simulink model "MCU_vectorControl_dsPIC33AK128MC106_MCLV_48V_300W_Float"  (R2024b)
settings: Solver=FixedStepDiscrete  StartTime=0.0  StopTime=10.0  FixedStep=50e-6  RelTol=1e-3  EnableMultiTasking=on
undefined symbols (not defined in the file or in its folder): A0, A4, ADC, B0, C10, C11, C6, C7, C8, control, D11, D12, DiscIntNeverNeededParam, inverter, Max, MaxPer, model, ms, NumBits1, NumBits2, P1, P17, P20, P39, P40, P41, P43, P44, P60, P61, Pin, PosRange1, PosRange2, PWM1_Trg1, Resol, s, Slope1, Slope2, us
libraries: simulink x35, MCHP_Blockset x22
(part 4 of 5)

== system MCU_vectorControl_dsPIC33AK128MC106_MCLV_48V_300W_Float/BOARD MCLV-48V-300W dsPIC33AK128MC106 MC DIM/ADC ==
  note: A5: IBUS
      | A7: VBUS
      | A11: Pot
  ADC HS 12b dsPICA1 : MCHP_Blockset/Analog IO/ADC HS 12b dsPICA  ADCREF=ADC 1 and ADC 2  ADC1_refChannel=0 (highest priority)  ADC2_refChannel=0 (highest priority)  ADC3_refChannel=Not used  ADC4_refChannel=Not used  ADC5_refChannel=Not used  CALRATE=once at startup  VREF_RNG=3.0V to 3.6V  BUFEN=off  info=0  SampleTime=1/Switching_Frequency  MCHP_PORT={ADC1_seq0.0}{ADC1A2}15:2:A2;{ADC2_seq0.0}{ADC2B0}15:2:B0;{ADC1_seq0.1}{ADC1B8}15:2:B8;{ADC2_seq0.1}{ADC2B9}15:2:B9;{ADC2_seq0.2}{ADC2A10}15:2:A10;{ADC1_seq0.0}{ADC1A2}15:2:A2;{ADC2_seq0.0}{ADC2B0}15:2:B0;{ADC1_seq0.1}{ADC1B8}15:2:B8;{ADC2_seq0.1}{ADC2B9}15:2:B9;{ADC2_seq0.2}{ADC2A10}15:2:A10;  MCHP_MASTERLINK=MCU_vectorControl_dsPIC33AK128MC106_MCLV_48V_300W_Flt/BOARD MCLV-48V-300W dsPIC33AK128MC106 MC DIM/Microchip Master  MCHP_CRC=34075787  ADC_Synchronisation=Triggered by custom source  ADC_Trig_TXT=PWM1_Trg1  ADC_TrigTimeStep=on  TrigSource_seq0_TXT=PWM1 adc trig 1  SampleTime_seq0_Tad_TXT="4.5 Tad  = 56.2ns  -  Rin < 5.2 kOhm"  ADC1_seq0_TXT=AD1 AN0 / A2 / Pin[12]  ADC1_seq0_align=Left aligned  ADC1_seq0_overSampling=x1 (12 bits)  ADC2_seq0_TXT=AD2 AN1 / B0 / Pin[20]  ADC2_seq0_align=Left aligned  ADC2_seq0_overSampling=x1 (12 bits)  ADC3_seq0_TXT="AD2 AN1 / B0 / Pin[20]  (L)"  ADC3_seq0_align=Right aligned  ADC3_seq0_overSampling=x1 (12 bits)  ADC4_seq0_TXT="AD2 AN1 / B0 / Pin[20]  (L)"  ADC4_seq0_align=Right aligned  ADC4_seq0_overSampling=x1 (12 bits)  ADC5_seq0_TXT="AD2 AN1 / B0 / Pin[20]  (L)"  ADC5_seq0_align=Right aligned  ADC5_seq0_overSampling=x1 (12 bits)  ADC1_seq0_1_TXT=AD1 AN11 / B8 / Pin[23]  ADC1_seq0_1_align=Left aligned  ADC1_seq0_1_overSampling=x1 (12 bits)  ADC2_seq0_1_TXT=AD2 AN10 / B9 / Pin[24]  ADC2_seq0_1_align=Left aligned  ADC2_seq0_1_overSampling=x1 (12 bits)  ADC3_seq0_1_TXT=Not Used  ADC3_seq0_1_align=Right aligned  ADC3_seq0_1_overSampling=x1 (12 bits)  ADC4_seq0_1_TXT=Not Used  ADC4_seq0_1_align=Right aligned  ADC4_seq0_1_overSampling=x1 (12 bits)  ADC5_seq0_1_TXT=Not Used  ADC5_seq0_1_align=Right aligned  ADC5_seq0_1_overSampling=x1 (12 bits)  ADC1_seq0_2_TXT=Not Used  ADC1_seq0_2_align=Right aligned  ADC1_seq0_2_overSampling=x1 (12 bits)  ADC2_seq0_2_TXT=AD2 AN7 / A10 / Pin[9]  ADC2_seq0_2_align=Left aligned  ADC2_seq0_2_overSampling=x1 (12 bits)  ADC3_seq0_2_TXT=Not Used  ADC3_seq0_2_align=Right aligned  ADC3_seq0_2_overSampling=x1 (12 bits)  ADC4_seq0_2_TXT=Not Used  ADC4_seq0_2_align=Right aligned  ADC4_seq0_2_overSampling=x1 (12 bits)  ADC5_seq0_2_TXT=Not Used  ADC5_seq0_2_align=Right aligned  ADC5_seq0_2_overSampling=x1 (12 bits)  ADC1_seq0_3_TXT=Not Used  ADC1_seq0_3_align=Right aligned  ADC1_seq0_3_overSampling=x1 (12 bits)  ADC2_seq0_3_TXT=Not Used  ADC2_seq0_3_align=Right aligned  ADC2_seq0_3_overSampling=x1 (12 bits)  ADC3_seq0_3_TXT=Not Used  ADC3_seq0_3_align=Right aligned  ADC3_seq0_3_overSampling=x1 (12 bits)  ADC4_seq0_3_TXT=Not Used  ADC4_seq0_3_align=Right aligned  ADC4_seq0_3_overSampling=x1 (12 bits)  ADC5_seq0_3_TXT=Not Used  ADC5_seq0_3_align=Right aligned  ADC5_seq0_3_overSampling=x1 (12 bits)  ADC1_seq0_4_TXT=Not Used  ADC1_seq0_4_align=Right aligned  ADC1_seq0_4_overSampling=x1 (12 bits)  ADC2_seq0_4_TXT=Not Used  ADC2_seq0_4_align=Right aligned  ADC2_seq0_4_overSampling=x1 (12 bits)  ADC3_seq0_4_TXT=Not Used  ADC3_seq0_4_align=Right aligned  ADC3_seq0_4_overSampling=x1 (12 bits)  ADC4_seq0_4_TXT=Not Used  ADC4_seq0_4_align=Right aligned  ADC4_seq0_4_overSampling=x1 (12 bits)  ADC5_seq0_4_TXT=Not Used  ADC5_seq0_4_align=Right aligned  ADC5_seq0_4_overSampling=x1 (12 bits)  ADC1_seq0_5_TXT=Not Used  ADC1_seq0_5_align=Right aligned  ADC1_seq0_5_overSampling=x1 (12 bits)  ADC2_seq0_5_TXT=Not Used  ADC2_seq0_5_align=Right aligned  ADC2_seq0_5_overSampling=x1 (12 bits)  ADC3_seq0_5_TXT=Not Used  ADC3_seq0_5_align=Right aligned  ADC3_seq0_5_overSampling=x1 (12 bits)  ADC4_seq0_5_TXT=Not Used  ADC4_seq0_5_align=Right aligned  ADC4_seq0_5_overSampling=x1 (12 bits)  ADC5_seq0_5_TXT=Not Used  ADC5_seq0_5_align=Right aligned  ADC5_seq0_5_overSampling=x1 (12 bits)  ADC_TRG2_ACCBRST_seq0=Burst - not interruptible  ADC1_NINSEL_seq0_TXT=Vss - single ended (unsigned)  ADC2_NINSEL_seq0_TXT=Vss - single ended (unsigned)  ADC3_NINSEL_seq0_TXT=Vss - single ended (unsigned)  ADC4_NINSEL_seq0_TXT=Vss - single ended (unsigned)  ADC5_NINSEL_seq0_TXT=Vss - single ended (unsigned)  TrigTimeStep_seq0=on  info_seq0=0  TrigSource_seq1_TXT=after previous sequence  SampleTime_seq1_Tad_TXT="0.5 Tad  = 6.25ns  -  Rin < 0 kOhm"  ADC1_seq1_TXT=Not Used  ADC1_seq1_align=Right aligned  ADC1_seq1_overSampling=x1 (12 bits)  ADC2_seq1_TXT=Not Used  ADC2_seq1_align=Right aligned  ADC2_seq1_overSampling=x1 (12 bits)  ADC3_seq1_TXT=Not Used  ADC3_seq1_align=Right aligned  ADC3_seq1_overSampling=x1 (12 bits)  ADC4_seq1_TXT=Not Used  ADC4_seq1_align=Right aligned  ADC4_seq1_overSampling=x1 (12 bits)  ADC5_seq1_TXT=Not Used  ADC5_seq1_align=Right aligned  ADC5_seq1_overSampling=x1 (12 bits)  ADC1_seq1_1_TXT=Not Used  ADC1_seq1_1_align=Right aligned  ADC1_seq1_1_overSampling=x1 (12 bits)  ADC2_seq1_1_TXT=Not Used  ADC2_seq1_1_align=Right aligned  ADC2_seq1_1_overSampling=x1 (12 bits)  ADC3_seq1_1_TXT=Not Used  ADC3_seq1_1_align=Right aligned  ADC3_seq1_1_overSampling=x1 (12 bits)  ADC4_seq1_1_TXT=Not Used  ADC4_seq1_1_align=Right aligned  ADC4_seq1_1_overSampling=x1 (12 bits)  ADC5_seq1_1_TXT=Not Used  ADC5_seq1_1_align=Right aligned  ADC5_seq1_1_overSampling=x1 (12 bits)  ADC1_seq1_2_TXT=Not Used  ADC1_seq1_2_align=Right aligned  ADC1_seq1_2_overSampling=x1 (12 bits)  ADC2_seq1_2_TXT=Not Used  ADC2_seq1_2_align=Right aligned  ADC2_seq1_2_overSampling=x1 (12 bits)  ADC3_seq1_2_TXT=Not Used  ADC3_seq1_2_align=Right aligned  ADC3_seq1_2_overSampling=x1 (12 bits)  ADC4_seq1_2_TXT=Not Used  ADC4_seq1_2_align=Right aligned  ADC4_seq1_2_overSampling=x1 (12 bits)  ADC5_seq1_2_TXT=Not Used  ADC5_seq1_2_align=Right aligned  ADC5_seq1_2_overSampling=x1 (12 bits)  ADC1_seq1_3_TXT=Not Used  ADC1_seq1_3_align=Right aligned  ADC1_seq1_3_overSampling=x1 (12 bits)  ADC2_seq1_3_TXT=Not Used  ADC2_seq1_3_align=Right aligned  ADC2_seq1_3_overSampling=x1 (12 bits)  ADC3_seq1_3_TXT=Not Used  ADC3_seq1_3_align=Right aligned  ADC3_seq1_3_overSampling=x1 (12 bits)  ADC4_seq1_3_TXT=Not Used  ADC4_seq1_3_align=Right aligned  ADC4_seq1_3_overSampling=x1 (12 bits)  ADC5_seq1_3_TXT=Not Used  ADC5_seq1_3_align=Right aligned  ADC5_seq1_3_overSampling=x1 (12 bits)  ADC1_seq1_4_TXT=Not Used  ADC1_seq1_4_align=Right aligned  ADC1_seq1_4_overSampling=x1 (12 bits)  ADC2_seq1_4_TXT=Not Used  ADC2_seq1_4_align=Right aligned  ADC2_seq1_4_overSampling=x1 (12 bits)  ADC3_seq1_4_TXT=Not Used  ADC3_seq1_4_align=Right aligned  ADC3_seq1_4_overSampling=x1 (12 bits)  ADC4_seq1_4_TXT=Not Used  ADC4_seq1_4_align=Right aligned  ADC4_seq1_4_overSampling=x1 (12 bits)  ADC5_seq1_4_TXT=Not Used  ADC5_seq1_4_align=Right aligned  ADC5_seq1_4_overSampling=x1 (12 bits)  ADC1_seq1_5_TXT=Not Used  ADC1_seq1_5_align=Right aligned  ADC1_seq1_5_overSampling=x1 (12 bits)  ADC2_seq1_5_TXT=Not Used  ADC2_seq1_5_align=Right aligned  ADC2_seq1_5_overSampling=x1 (12 bits)  ADC3_seq1_5_TXT=Not Used  ADC3_seq1_5_align=Right aligned  ADC3_seq1_5_overSampling=x1 (12 bits)  ADC4_seq1_5_TXT=Not Used  ADC4_seq1_5_align=Right aligned  ADC4_seq1_5_overSampling=x1 (12 bits)  ADC5_seq1_5_TXT=Not Used  ADC5_seq1_5_align=Right aligned  ADC5_seq1_5_overSampling=x1 (12 bits)  ADC_TRG2_ACCBRST_seq1=Burst - not interruptible  ADC1_NINSEL_seq1_TXT=Vss - single ended (unsigned)  ADC2_NINSEL_seq1_TXT=Vss - single ended (unsigned)  ADC3_NINSEL_seq1_TXT=Vss - single ended (unsigned)  ADC4_NINSEL_seq1_TXT=Vss - single ended (unsigned)  ADC5_NINSEL_seq1_TXT=Vss - single ended (unsigned)  TrigTimeStep_seq1=off  info_seq1=0  TrigSource_seq2_TXT=after previous sequence  SampleTime_seq2_Tad_TXT="0.5 Tad  = 6.25ns  -  Rin < 0 kOhm"  ADC1_seq2_TXT=Not Used  ADC1_seq2_align=Right aligned  ADC1_seq2_overSampling=x1 (12 bits)  ADC2_seq2_TXT=Not Used  ADC2_seq2_align=Right aligned  ADC2_seq2_overSampling=x1 (12 bits)  ADC3_seq2_TXT=Not Used  ADC3_seq2_align=Right aligned  ADC3_seq2_overSampling=x1 (12 bits)  ADC4_seq2_TXT=Not Used  ADC4_seq2_align=Right aligned  ADC4_seq2_overSampling=x1 (12 bits)  ADC5_seq2_TXT=Not Used  ADC5_seq2_align=Right aligned  ADC5_seq2_overSampling=x1 (12 bits)  ADC1_seq2_1_TXT=Not Used  ADC1_seq2_1_align=Right aligned  ADC1_seq2_1_overSampling=x1 (12 bits)  ADC2_seq2_1_TXT=Not Used  ADC2_seq2_1_align=Right aligned  ADC2_seq2_1_overSampling=x1 (12 bits)  ADC3_seq2_1_TXT=Not Used  ADC3_seq2_1_align=Right aligned  ADC3_seq2_1_overSampling=x1 (12 bits)  ADC4_seq2_1_TXT=Not Used  ADC4_seq2_1_align=Right aligned  ADC4_seq2_1_overSampling=x1 (12 bits)  ADC5_seq2_1_TXT=Not Used  ADC5_seq2_1_align=Right aligned  ADC5_seq2_1_overSampling=x1 (12 bits)  ADC1_seq2_2_TXT=Not Used  ADC1_seq2_2_align=Right aligned  ADC1_seq2_2_overSampling=x1 (12 bits)  ADC2_seq2_2_TXT=Not Used  ADC2_seq2_2_align=Right aligned  ADC2_seq2_2_overSampling=x1 (12 bits)  ADC3_seq2_2_TXT=Not Used  ADC3_seq2_2_align=Right aligned  ADC3_seq2_2_overSampling=x1 (12 bits)  ADC4_seq2_2_TXT=Not Used  ADC4_seq2_2_align=Right aligned  ADC4_seq2_2_overSampling=x1 (12 bits)  ADC5_seq2_2_TXT=Not Used  ADC5_seq2_2_align=Right aligned  ADC5_seq2_2_overSampling=x1 (12 bits)  ADC1_seq2_3_TXT=Not Used  ADC1_seq2_3_align=Right aligned  ADC1_seq2_3_overSampling=x1 (12 bits)  ADC2_seq2_3_TXT=Not Used  ADC2_seq2_3_align=Right aligned  ADC2_seq2_3_overSampling=x1 (12 bits)  ADC3_seq2_3_TXT=Not Used  ADC3_seq2_3_align=Right aligned  ADC3_seq2_3_overSampling=x1 (12 bits)  ADC4_seq2_3_TXT=Not Used  ADC4_seq2_3_align=Right aligned  ADC4_seq2_3_overSampling=x1 (12 bits)  ADC5_seq2_3_TXT=Not Used  ADC5_seq2_3_align=Right aligned  ADC5_seq2_3_overSampling=x1 (12 bits)  ADC1_seq2_4_TXT=Not Used  ADC1_seq2_4_align=Right aligned  ADC1_seq2_4_overSampling=x1 (12 bits)  ADC2_seq2_4_TXT=Not Used  ADC2_seq2_4_align=Right aligned  ADC2_seq2_4_overSampling=x1 (12 bits)  ADC3_seq2_4_TXT=Not Used  ADC3_seq2_4_align=Right aligned  ADC3_seq2_4_overSampling=x1 (12 bits)  ADC4_seq2_4_TXT=Not Used  ADC4_seq2_4_align=Right aligned  ADC4_seq2_4_overSampling=x1 (12 bits)  ADC5_seq2_4_TXT=Not Used  ADC5_seq2_4_align=Right aligned  ADC5_seq2_4_overSampling=x1 (12 bits)  ADC1_seq2_5_TXT=Not Used  ADC1_seq2_5_align=Right aligned  ADC1_seq2_5_overSampling=x1 (12 bits)  ADC2_seq2_5_TXT=Not Used  ADC2_seq2_5_align=Right aligned  ADC2_seq2_5_overSampling=x1 (12 bits)  ADC3_seq2_5_TXT=Not Used  ADC3_seq2_5_align=Right aligned  ADC3_seq2_5_overSampling=x1 (12 bits)  ADC4_seq2_5_TXT=Not Used  ADC4_seq2_5_align=Right aligned  ADC4_seq2_5_overSampling=x1 (12 bits)  ADC5_seq2_5_TXT=Not Used  ADC5_seq2_5_align=Right aligned  ADC5_seq2_5_overSampling=x1 (12 bits)  ADC_TRG2_ACCBRST_seq2=Burst - not interruptible  ADC1_NINSEL_seq2_TXT=Vss - single ended (unsigned)  ADC2_NINSEL_seq2_TXT=Vss - single ended (unsigned)  ADC3_NINSEL_seq2_TXT=Vss - single ended (unsigned)  ADC4_NINSEL_seq2_TXT=Vss - single ended (unsigned)  ADC5_NINSEL_seq2_TXT=Vss - single ended (unsigned)  TrigTimeStep_seq2=off  info_seq2=0  TrigSource_seq3_TXT=after previous sequence  SampleTime_seq3_Tad_TXT="0.5 Tad  = 6.25ns  -  Rin < 0 kOhm"  ADC1_seq3_TXT=Not Used  ADC1_seq3_align=Right aligned  ADC1_seq3_overSampling=x1 (12 bits)  ADC2_seq3_TXT=Not Used  ADC2_seq3_align=Right aligned  ADC2_seq3_overSampling=x1 (12 bits)  ADC3_seq3_TXT=Not Used  ADC3_seq3_align=Right aligned  ADC3_seq3_overSampling=x1 (12 bits)  ADC4_seq3_TXT=Not Used  ADC4_seq3_align=Right aligned  ADC4_seq3_overSampling=x1 (12 bits)  ADC5_seq3_TXT=Not Used  ADC5_seq3_align=Right aligned  ADC5_seq3_overSampling=x1 (12 bits)  ADC1_seq3_1_TXT=Not Used  ADC1_seq3_1_align=Right aligned  ADC1_seq3_1_overSampling=x1 (12 bits)  ADC2_seq3_1_TXT=Not Used  ADC2_seq3_1_align=Right aligned  ADC2_seq3_1_overSampling=x1 (12 bits)  ADC3_seq3_1_TXT=Not Used  ADC3_seq3_1_align=Right aligned  ADC3_seq3_1_overSampling=x1 (12 bits)  ADC4_seq3_1_TXT=Not Used  ADC4_seq3_1_align=Right aligned  ADC4_seq3_1_overSampling=x1 (12 bits)  ADC5_seq3_1_TXT=Not Used  ADC5_seq3_1_align=Right aligned  ADC5_seq3_1_overSampling=x1 (12 bits)  ADC1_seq3_2_TXT=Not Used  ADC1_seq3_2_align=Right aligned  ADC1_seq3_2_overSampling=x1 (12 bits)  ADC2_seq3_2_TXT=Not Used  ADC2_seq3_2_align=Right aligned  ADC2_seq3_2_overSampling=x1 (12 bits)  ADC3_seq3_2_TXT=Not Used  ADC3_seq3_2_align=Right aligned  ADC3_seq3_2_overSampling=x1 (12 bits)  ADC4_seq3_2_TXT=Not Used  ADC4_seq3_2_align=Right aligned  ADC4_seq3_2_overSampling=x1 (12 bits)  ADC5_seq3_2_TXT=Not Used  ADC5_seq3_2_align=Right aligned  ADC5_seq3_2_overSampling=x1 (12 bits)  ADC1_seq3_3_TXT=Not Used  ADC1_seq3_3_align=Right aligned  ADC1_seq3_3_overSampling=x1 (12 bits)  ADC2_seq3_3_TXT=Not Used  ADC2_seq3_3_align=Right aligned  ADC2_seq3_3_overSampling=x1 (12 bits)  ADC3_seq3_3_TXT=Not Used  ADC3_seq3_3_align=Right aligned  ADC3_seq3_3_overSampling=x1 (12 bits)  ADC4_seq3_3_TXT=Not Used  ADC4_seq3_3_align=Right aligned  ADC4_seq3_3_overSampling=x1 (12 bits)  ADC5_seq3_3_TXT=Not Used  ADC5_seq3_3_align=Right aligned  ADC5_seq3_3_overSampling=x1 (12 bits)  ADC1_seq3_4_TXT=Not Used  ADC1_seq3_4_align=Right aligned  ADC1_seq3_4_overSampling=x1 (12 bits)  ADC2_seq3_4_TXT=Not Used  ADC2_seq3_4_align=Right aligned  ADC2_seq3_4_overSampling=x1 (12 bits)  ADC3_seq3_4_TXT=Not Used  ADC3_seq3_4_align=Right aligned  ADC3_seq3_4_overSampling=x1 (12 bits)  ADC4_seq3_4_TXT=Not Used  ADC4_seq3_4_align=Right aligned  ADC4_seq3_4_overSampling=x1 (12 bits)  ADC5_seq3_4_TXT=Not Used  ADC5_seq3_4_align=Right aligned  ADC5_seq3_4_overSampling=x1 (12 bits)  ADC1_seq3_5_TXT=Not Used  ADC1_seq3_5_align=Right aligned  ADC1_seq3_5_overSampling=x1 (12 bits)  ADC2_seq3_5_TXT=Not Used  ADC2_seq3_5_align=Right aligned  ADC2_seq3_5_overSampling=x1 (12 bits)  ADC3_seq3_5_TXT=Not Used  ADC3_seq3_5_align=Right aligned  ADC3_seq3_5_overSampling=x1 (12 bits)  ADC4_seq3_5_TXT=Not Used  ADC4_seq3_5_align=Right aligned  ADC4_seq3_5_overSampling=x1 (12 bits)  ADC5_seq3_5_TXT=Not Used  ADC5_seq3_5_align=Right aligned  ADC5_seq3_5_overSampling=x1 (12 bits)  ADC_TRG2_ACCBRST_seq3=Burst - not interruptible  ADC1_NINSEL_seq3_TXT=Vss - single ended (unsigned)  ADC2_NINSEL_seq3_TXT=Vss - single ended (unsigned)  ADC3_NINSEL_seq3_TXT=Vss - single ended (unsigned)  ADC4_NINSEL_seq3_TXT=Vss - single ended (unsigned)  ADC5_NINSEL_seq3_TXT=Vss - single ended (unsigned)  TrigTimeStep_seq3=off  info_seq3=0  TrigSource_seq4_TXT=after previous sequence  SampleTime_seq4_Tad_TXT="0.5 Tad  = 6.25ns  -  Rin < 0 kOhm"  ADC1_seq4_TXT=Not Used  ADC1_seq4_align=Right aligned  ADC1_seq4_overSampling=x1 (12 bits)  ADC2_seq4_TXT=Not Used  ADC2_seq4_align=Right aligned  ADC2_seq4_overSampling=x1 (12 bits)  ADC3_seq4_TXT=Not Used  ADC3_seq4_align=Right aligned  ADC3_seq4_overSampling=x1 (12 bits)  ADC4_seq4_TXT=Not Used  ADC4_seq4_align=Right aligned  ADC4_seq4_overSampling=x1 (12 bits)  ADC5_seq4_TXT=Not Used  ADC5_seq4_align=Right aligned  ADC5_seq4_overSampling=x1 (12 bits)  ADC1_seq4_1_TXT=Not Used  ADC1_seq4_1_align=Right aligned  ADC1_seq4_1_overSampling=x1 (12 bits)  ADC2_seq4_1_TXT=Not Used  ADC2_seq4_1_align=Right aligned  ADC2_seq4_1_overSampling=x1 (12 bits)  ADC3_seq4_1_TXT=Not Used  ADC3_seq4_1_align=Right aligned  ADC3_seq4_1_overSampling=x1 (12 bits)  ADC4_seq4_1_TXT=Not Used  ADC4_seq4_1_align=Right aligned  ADC4_seq4_1_overSampling=x1 (12 bits)  ADC5_seq4_1_TXT=Not Used  ADC5_seq4_1_align=Right aligned  ADC5_seq4_1_overSampling=x1 (12 bits)  ADC1_seq4_2_TXT=Not Used  ADC1_seq4_2_align=Right aligned  ADC1_seq4_2_overSampling=x1 (12 bits)  ADC2_seq4_2_TXT=Not Used  ADC2_seq4_2_align=Right aligned  ADC2_seq4_2_overSampling=x1 (12 bits)  ADC3_seq4_2_TXT=Not Used  ADC3_seq4_2_align=Right aligned  ADC3_seq4_2_overSampling=x1 (12 bits)  ADC4_seq4_2_TXT=Not Used  ADC4_seq4_2_align=Right aligned  ADC4_seq4_2_overSampling=x1 (12 bits)  ADC5_seq4_2_TXT=Not Used  ADC5_seq4_2_align=Right aligned  ADC5_seq4_2_overSampling=x1 (12 bits)  ADC1_seq4_3_TXT=Not Used  ADC1_seq4_3_align=Right aligned  ADC1_seq4_3_overSampling=x1 (12 bits)  ADC2_seq4_3_TXT=Not Used  ADC2_seq4_3_align=Right aligned  ADC2_seq4_3_overSampling=x1 (12 bits)  ADC3_seq4_3_TXT=Not Used  ADC3_seq4_3_align=Right aligned  ADC3_seq4_3_overSampling=x1 (12 bits)  ADC4_seq4_3_TXT=Not Used  ADC4_seq4_3_align=Right aligned  ADC4_seq4_3_overSampling=x1 (12 bits)  ADC5_seq4_3_TXT=Not Used  ADC5_seq4_3_align=Right aligned  ADC5_seq4_3_overSampling=x1 (12 bits)  ADC1_seq4_4_TXT=Not Used  ADC1_seq4_4_align=Right aligned  ADC1_seq4_4_overSampling=x1 (12 bits)  ADC2_seq4_4_TXT=Not Used  ADC2_seq4_4_align=Right aligned  ADC2_seq4_4_overSampling=x1 (12 bits)  ADC3_seq4_4_TXT=Not Used  ADC3_seq4_4_align=Right aligned  ADC3_seq4_4_overSampling=x1 (12 bits)  ADC4_seq4_4_TXT=Not Used  ADC4_seq4_4_align=Right aligned  ADC4_seq4_4_overSampling=x1 (12 bits)  ADC5_seq4_4_TXT=Not Used  ADC5_seq4_4_align=Right aligned  ADC5_seq4_4_overSampling=x1 (12 bits)  ADC1_seq4_5_TXT=Not Used  ADC1_seq4_5_align=Right aligned  ADC1_seq4_5_overSampling=x1 (12 bits)  ADC2_seq4_5_TXT=Not Used  ADC2_seq4_5_align=Right aligned  ADC2_seq4_5_overSampling=x1 (12 bits)  ADC3_seq4_5_TXT=Not Used  ADC3_seq4_5_align=Right aligned  ADC3_seq4_5_overSampling=x1 (12 bits)  ADC4_seq4_5_TXT=Not Used  ADC4_seq4_5_align=Right aligned  ADC4_seq4_5_overSampling=x1 (12 bits)  ADC5_seq4_5_TXT=Not Used  ADC5_seq4_5_align=Right aligned  ADC5_seq4_5_overSampling=x1 (12 bits)  ADC_TRG2_ACCBRST_seq4=Burst - not interruptible  ADC1_NINSEL_seq4_TXT=Vss - single ended (unsigned)  ADC2_NINSEL_seq4_TXT=Vss - single ended (unsigned)  ADC3_NINSEL_seq4_TXT=Vss - single ended (unsigned)  ADC4_NINSEL_seq4_TXT=Vss - single ended (unsigned)  ADC5_NINSEL_seq4_TXT=Vss - single ended (unsigned)  TrigTimeStep_seq4=off  info_seq4=0  TrigSource_seq5_TXT=after previous sequence  SampleTime_seq5_Tad_TXT="0.5 Tad  = 6.25ns  -  Rin < 0 kOhm"  ADC1_seq5_TXT=Not Used  ADC1_seq5_align=Right aligned  ADC1_seq5_overSampling=x1 (12 bits)  ADC2_seq5_TXT=Not Used  ADC2_seq5_align=Right aligned  ADC2_seq5_overSampling=x1 (12 bits)  ADC3_seq5_TXT=Not Used  ADC3_seq5_align=Right aligned  ADC3_seq5_overSampling=x1 (12 bits)  ADC4_seq5_TXT=Not Used  ADC4_seq5_align=Right aligned  ADC4_seq5_overSampling=x1 (12 bits)  ADC5_seq5_TXT=Not Used  ADC5_seq5_align=Right aligned  ADC5_seq5_overSampling=x1 (12 bits)  ADC1_seq5_1_TXT=Not Used  ADC1_seq5_1_align=Right aligned  ADC1_seq5_1_overSampling=x1 (12 bits)  ADC2_seq5_1_TXT=Not Used  ADC2_seq5_1_align=Right aligned  ADC2_seq5_1_overSampling=x1 (12 bits)  ADC3_seq5_1_TXT=Not Used  ADC3_seq5_1_align=Right aligned  ADC3_seq5_1_overSampling=x1 (12 bits)  ADC4_seq5_1_TXT=Not Used  ADC4_seq5_1_align=Right aligned  ADC4_seq5_1_overSampling=x1 (12 bits)  ADC5_seq5_1_TXT=Not Used  ADC5_seq5_1_align=Right aligned  ADC5_seq5_1_overSampling=x1 (12 bits)  ADC1_seq5_2_TXT=Not Used  ADC1_seq5_2_align=Right aligned  ADC1_seq5_2_overSampling=x1 (12 bits)  ADC2_seq5_2_TXT=Not Used  ADC2_seq5_2_align=Right aligned  ADC2_seq5_2_overSampling=x1 (12 bits)  ADC3_seq5_2_TXT=Not Used  ADC3_seq5_2_align=Right aligned  ADC3_seq5_2_overSampling=x1 (12 bits)  ADC4_seq5_2_TXT=Not Used  ADC4_seq5_2_align=Right aligned  ADC4_seq5_2_overSampling=x1 (12 bits)  ADC5_seq5_2_TXT=Not Used  ADC5_seq5_2_align=Right aligned  ADC5_seq5_2_overSampling=x1 (12 bits)  ADC1_seq5_3_TXT=Not Used  ADC1_seq5_3_align=Right aligned  ADC1_seq5_3_overSampling=x1 (12 bits)  ADC2_seq5_3_TXT=Not Used  ADC2_seq5_3_align=Right aligned  ADC2_seq5_3_overSampling=x1 (12 bits)  ADC3_seq5_3_TXT=Not Used  ADC3_seq5_3_align=Right aligned  ADC3_seq5_3_overSampling=x1 (12 bits)  ADC4_seq5_3_TXT=Not Used  ADC4_seq5_3_align=Right aligned  ADC4_seq5_3_overSampling=x1 (12 bits)  ADC5_seq5_3_TXT=Not Used  ADC5_seq5_3_align=Right aligned  ADC5_seq5_3_overSampling=x1 (12 bits)  ADC1_seq5_4_TXT=Not Used  ADC1_seq5_4_align=Right aligned  ADC1_seq5_4_overSampling=x1 (12 bits)  ADC2_seq5_4_TXT=Not Used  ADC2_seq5_4_align=Right aligned  ADC2_seq5_4_overSampling=x1 (12 bits)  ADC3_seq5_4_TXT=Not Used  ADC3_seq5_4_align=Right aligned  ADC3_seq5_4_overSampling=x1 (12 bits)  ADC4_seq5_4_TXT=Not Used  ADC4_seq5_4_align=Right aligned  ADC4_seq5_4_overSampling=x1 (12 bits)  ADC5_seq5_4_TXT=Not Used  ADC5_seq5_4_align=Right aligned  ADC5_seq5_4_overSampling=x1 (12 bits)  ADC1_seq5_5_TXT=Not Used  ADC1_seq5_5_align=Right aligned  ADC1_seq5_5_overSampling=x1 (12 bits)  ADC2_seq5_5_TXT=Not Used  ADC2_seq5_5_align=Right aligned  ADC2_seq5_5_overSampling=x1 (12 bits)  ADC3_seq5_5_TXT=Not Used  ADC3_seq5_5_align=Right aligned  ADC3_seq5_5_overSampling=x1 (12 bits)  ADC4_seq5_5_TXT=Not Used  ADC4_seq5_5_align=Right aligned  ADC4_seq5_5_overSampling=x1 (12 bits)  ADC5_seq5_5_TXT=Not Used  ADC5_seq5_5_align=Right aligned  ADC5_seq5_5_overSampling=x1 (12 bits)  ADC_TRG2_ACCBRST_seq5=Burst - not interruptible  ADC1_NINSEL_seq5_TXT=Vss - single ended (unsigned)  ADC2_NINSEL_seq5_TXT=Vss - single ended (unsigned)  ADC3_NINSEL_seq5_TXT=Vss - single ended (unsigned)  ADC4_NINSEL_seq5_TXT=Vss - single ended (unsigned)  ADC5_NINSEL_seq5_TXT=Vss - single ended (unsigned)  TrigTimeStep_seq5=off  info_seq5=0
      settings: SourceProductName=MPLAB Device Blocks for Simulink
  ADC HS 12b dsPICA2 : MCHP_Blockset/Analog IO/ADC HS 12b dsPICA  ADCREF=ADC 1  ADC1_refChannel=5  ADC2_refChannel=5  ADC3_refChannel=Not used  ADC4_refChannel=Not used  ADC5_refChannel=Not used  CALRATE=once at startup  VREF_RNG=3.0V to 3.6V  BUFEN=off  info=0  SampleTime=1/Switching_Frequency  MCHP_PORT={ADC1_seq0.0}{ADC1A5}15:2:A5;{ADC1_seq0.1}{ADC1A7}15:2:A7;{ADC1_seq0.2}{ADC1A11}15:2:A11;{ADC1_seq0.0}{ADC1A5}15:2:A5;{ADC1_seq0.1}{ADC1A7}15:2:A7;{ADC1_seq0.2}{ADC1A11}15:2:A11;  MCHP_MASTERLINK=MCU_vectorControl_dsPIC33AK128MC106_MCLV_48V_300W_Flt/BOARD MCLV-48V-300W dsPIC33AK128MC106 MC DIM/Microchip Master  MCHP_CRC=33984699  ADC_Synchronisation=off  ADC_Trig_TXT=off  ADC_TrigTimeStep=off  TrigSource_seq0_TXT=PWM1 adc trig 1  SampleTime_seq0_Tad_TXT="8.5 Tad  = 106ns  -  Rin < 11 kOhm"  ADC1_seq0_TXT=AD1 AN3 / A5 / Pin[15]  ADC1_seq0_align=Left aligned  ADC1_seq0_overSampling=x1 (12 bits)  ADC2_seq0_TXT=Not Used  ADC2_seq0_align=Right aligned  ADC2_seq0_overSampling=x1 (12 bits)  ADC3_seq0_TXT="AD2 AN1 / B0 / Pin[20]  (L)"  ADC3_seq0_align=Right aligned  ADC3_seq0_overSampling=x1 (12 bits)  ADC4_seq0_TXT="AD2 AN1 / B0 / Pin[20]  (L)"  ADC4_seq0_align=Right aligned  ADC4_seq0_overSampling=x1 (12 bits)  ADC5_seq0_TXT="AD2 AN1 / B0 / Pin[20]  (L)"  ADC5_seq0_align=Right aligned  ADC5_seq0_overSampling=x1 (12 bits)  ADC1_seq0_1_TXT=AD1 AN6 / A7 / Pin[2]  ADC1_seq0_1_align=Left aligned  ADC1_seq0_1_overSampling=x1 (12 bits)  ADC2_seq0_1_TXT=Not Used  ADC2_seq0_1_align=Right aligned  ADC2_seq0_1_overSampling=x1 (12 bits)  ADC3_seq0_1_TXT=Not Used  ADC3_seq0_1_align=Right aligned  ADC3_seq0_1_overSampling=x1 (12 bits)  ADC4_seq0_1_TXT=Not Used  ADC4_seq0_1_align=Right aligned  ADC4_seq0_1_overSampling=x1 (12 bits)  ADC5_seq0_1_TXT=Not Used  ADC5_seq0_1_align=Right aligned  ADC5_seq0_1_overSampling=x1 (12 bits)  ADC1_seq0_2_TXT=AD1 AN10 / A11 / Pin[6]  ADC1_seq0_2_align=Left aligned  ADC1_seq0_2_overSampling=x1 (12 bits)  ADC2_seq0_2_TXT=Not Used  ADC2_seq0_2_align=Right aligned  ADC2_seq0_2_overSampling=x1 (12 bits)  ADC3_seq0_2_TXT=Not Used  ADC3_seq0_2_align=Right aligned  ADC3_seq0_2_overSampling=x1 (12 bits)  ADC4_seq0_2_TXT=Not Used  ADC4_seq0_2_align=Right aligned  ADC4_seq0_2_overSampling=x1 (12 bits)  ADC5_seq0_2_TXT=Not Used  ADC5_seq0_2_align=Right aligned  ADC5_seq0_2_overSampling=x1 (12 bits)  ADC1_seq0_3_TXT=Not Used  ADC1_seq0_3_align=Right aligned  ADC1_seq0_3_overSampling=x1 (12 bits)  ADC2_seq0_3_TXT=Not Used  ADC2_seq0_3_align=Right aligned  ADC2_seq0_3_overSampling=x1 (12 bits)  ADC3_seq0_3_TXT=Not Used  ADC3_seq0_3_align=Right aligned  ADC3_seq0_3_overSampling=x1 (12 bits)  ADC4_seq0_3_TXT=Not Used  ADC4_seq0_3_align=Right aligned  ADC4_seq0_3_overSampling=x1 (12 bits)  ADC5_seq0_3_TXT=Not Used  ADC5_seq0_3_align=Right aligned  ADC5_seq0_3_overSampling=x1 (12 bits)  ADC1_seq0_4_TXT=Not Used  ADC1_seq0_4_align=Right aligned  ADC1_seq0_4_overSampling=x1 (12 bits)  ADC2_seq0_4_TXT=Not Used  ADC2_seq0_4_align=Right aligned  ADC2_seq0_4_overSampling=x1 (12 bits)  ADC3_seq0_4_TXT=Not Used  ADC3_seq0_4_align=Right aligned  ADC3_seq0_4_overSampling=x1 (12 bits)  ADC4_seq0_4_TXT=Not Used  ADC4_seq0_4_align=Right aligned  ADC4_seq0_4_overSampling=x1 (12 bits)  ADC5_seq0_4_TXT=Not Used  ADC5_seq0_4_align=Right aligned  ADC5_seq0_4_overSampling=x1 (12 bits)  ADC1_seq0_5_TXT=Not Used  ADC1_seq0_5_align=Right aligned  ADC1_seq0_5_overSampling=x1 (12 bits)  ADC2_seq0_5_TXT=Not Used  ADC2_seq0_5_align=Right aligned  ADC2_seq0_5_overSampling=x1 (12 bits)  ADC3_seq0_5_TXT=Not Used  ADC3_seq0_5_align=Right aligned  ADC3_seq0_5_overSampling=x1 (12 bits)  ADC4_seq0_5_TXT=Not Used  ADC4_seq0_5_align=Right aligned  ADC4_seq0_5_overSampling=x1 (12 bits)  ADC5_seq0_5_TXT=Not Used  ADC5_seq0_5_align=Right aligned  ADC5_seq0_5_overSampling=x1 (12 bits)  ADC_TRG2_ACCBRST_seq0=Burst - not interruptible  ADC1_NINSEL_seq0_TXT=Vss - single ended (unsigned)  ADC2_NINSEL_seq0_TXT=Vss - single ended (unsigned)  ADC3_NINSEL_seq0_TXT=Vss - single ended (unsigned)  ADC4_NINSEL_seq0_TXT=Vss - single ended (unsigned)  ADC5_NINSEL_seq0_TXT=Vss - single ended (unsigned)  TrigTimeStep_seq0=off  info_seq0=0  TrigSource_seq1_TXT=after previous sequence  SampleTime_seq1_Tad_TXT="0.5 Tad  = 6.25ns  -  Rin < 0 kOhm"  ADC1_seq1_TXT=Not Used  ADC1_seq1_align=Right aligned  ADC1_seq1_overSampling=x1 (12 bits)  ADC2_seq1_TXT=Not Used  ADC2_seq1_align=Right aligned  ADC2_seq1_overSampling=x1 (12 bits)  ADC3_seq1_TXT=Not Used  ADC3_seq1_align=Right aligned  ADC3_seq1_overSampling=x1 (12 bits)  ADC4_seq1_TXT=Not Used  ADC4_seq1_align=Right aligned  ADC4_seq1_overSampling=x1 (12 bits)  ADC5_seq1_TXT=Not Used  ADC5_seq1_align=Right aligned  ADC5_seq1_overSampling=x1 (12 bits)  ADC1_seq1_1_TXT=Not Used  ADC1_seq1_1_align=Right aligned  ADC1_seq1_1_overSampling=x1 (12 bits)  ADC2_seq1_1_TXT=Not Used  ADC2_seq1_1_align=Right aligned  ADC2_seq1_1_overSampling=x1 (12 bits)  ADC3_seq1_1_TXT=Not Used  ADC3_seq1_1_align=Right aligned  ADC3_seq1_1_overSampling=x1 (12 bits)  ADC4_seq1_1_TXT=Not Used  ADC4_seq1_1_align=Right aligned  ADC4_seq1_1_overSampling=x1 (12 bits)  ADC5_seq1_1_TXT=Not Used  ADC5_seq1_1_align=Right aligned  ADC5_seq1_1_overSampling=x1 (12 bits)  ADC1_seq1_2_TXT=Not Used  ADC1_seq1_2_align=Right aligned  ADC1_seq1_2_overSampling=x1 (12 bits)  ADC2_seq1_2_TXT=Not Used  ADC2_seq1_2_align=Right aligned  ADC2_seq1_2_overSampling=x1 (12 bits)  ADC3_seq1_2_TXT=Not Used  ADC3_seq1_2_align=Right aligned  ADC3_seq1_2_overSampling=x1 (12 bits)  ADC4_seq1_2_TXT=Not Used  ADC4_seq1_2_align=Right aligned  ADC4_seq1_2_overSampling=x1 (12 bits)  ADC5_seq1_2_TXT=Not Used  ADC5_seq1_2_align=Right aligned  ADC5_seq1_2_overSampling=x1 (12 bits)  ADC1_seq1_3_TXT=Not Used  ADC1_seq1_3_align=Right aligned  ADC1_seq1_3_overSampling=x1 (12 bits)  ADC2_seq1_3_TXT=Not Used  ADC2_seq1_3_align=Right aligned  ADC2_seq1_3_overSampling=x1 (12 bits)  ADC3_seq1_3_TXT=Not Used  ADC3_seq1_3_align=Right aligned  ADC3_seq1_3_overSampling=x1 (12 bits)  ADC4_seq1_3_TXT=Not Used  ADC4_seq1_3_align=Right aligned  ADC4_seq1_3_overSampling=x1 (12 bits)  ADC5_seq1_3_TXT=Not Used  ADC5_seq1_3_align=Right aligned  ADC5_seq1_3_overSampling=x1 (12 bits)  ADC1_seq1_4_TXT=Not Used  ADC1_seq1_4_align=Right aligned  ADC1_seq1_4_overSampling=x1 (12 bits)  ADC2_seq1_4_TXT=Not Used  ADC2_seq1_4_align=Right aligned  ADC2_seq1_4_overSampling=x1 (12 bits)  ADC3_seq1_4_TXT=Not Used  ADC3_seq1_4_align=Right aligned  ADC3_seq1_4_overSampling=x1 (12 bits)  ADC4_seq1_4_TXT=Not Used  ADC4_seq1_4_align=Right aligned  ADC4_seq1_4_overSampling=x1 (12 bits)  ADC5_seq1_4_TXT=Not Used  ADC5_seq1_4_align=Right aligned  ADC5_seq1_4_overSampling=x1 (12 bits)  ADC1_seq1_5_TXT=Not Used  ADC1_seq1_5_align=Right aligned  ADC1_seq1_5_overSampling=x1 (12 bits)  ADC2_seq1_5_TXT=Not Used  ADC2_seq1_5_align=Right aligned  ADC2_seq1_5_overSampling=x1 (12 bits)  ADC3_seq1_5_TXT=Not Used  ADC3_seq1_5_align=Right aligned  ADC3_seq1_5_overSampling=x1 (12 bits)  ADC4_seq1_5_TXT=Not Used  ADC4_seq1_5_align=Right aligned  ADC4_seq1_5_overSampling=x1 (12 bits)  ADC5_seq1_5_TXT=Not Used  ADC5_seq1_5_align=Right aligned  ADC5_seq1_5_overSampling=x1 (12 bits)  ADC_TRG2_ACCBRST_seq1=Burst - not interruptible  ADC1_NINSEL_seq1_TXT=Vss - single ended (unsigned)  ADC2_NINSEL_seq1_TXT=Vss - single ended (unsigned)  ADC3_NINSEL_seq1_TXT=Vss - single ended (unsigned)  ADC4_NINSEL_seq1_TXT=Vss - single ended (unsigned)  ADC5_NINSEL_seq1_TXT=Vss - single ended (unsigned)  TrigTimeStep_seq1=off  info_seq1=0  TrigSource_seq2_TXT=after previous sequence  SampleTime_seq2_Tad_TXT="0.5 Tad  = 6.25ns  -  Rin < 0 kOhm"  ADC1_seq2_TXT=Not Used  ADC1_seq2_align=Right aligned  ADC1_seq2_overSampling=x1 (12 bits)  ADC2_seq2_TXT=Not Used  ADC2_seq2_align=Right aligned  ADC2_seq2_overSampling=x1 (12 bits)  ADC3_seq2_TXT=Not Used  ADC3_seq2_align=Right aligned  ADC3_seq2_overSampling=x1 (12 bits)  ADC4_seq2_TXT=Not Used  ADC4_seq2_align=Right aligned  ADC4_seq2_overSampling=x1 (12 bits)  ADC5_seq2_TXT=Not Used  ADC5_seq2_align=Right aligned  ADC5_seq2_overSampling=x1 (12 bits)  ADC1_seq2_1_TXT=Not Used  ADC1_seq2_1_align=Right aligned  ADC1_seq2_1_overSampling=x1 (12 bits)  ADC2_seq2_1_TXT=Not Used  ADC2_seq2_1_align=Right aligned  ADC2_seq2_1_overSampling=x1 (12 bits)  ADC3_seq2_1_TXT=Not Used  ADC3_seq2_1_align=Right aligned  ADC3_seq2_1_overSampling=x1 (12 bits)  ADC4_seq2_1_TXT=Not Used  ADC4_seq2_1_align=Right aligned  ADC4_seq2_1_overSampling=x1 (12 bits)  ADC5_seq2_1_TXT=Not Used  ADC5_seq2_1_align=Right aligned  ADC5_seq2_1_overSampling=x1 (12 bits)  ADC1_seq2_2_TXT=Not Used  ADC1_seq2_2_align=Right aligned  ADC1_seq2_2_overSampling=x1 (12 bits)  ADC2_seq2_2_TXT=Not Used  ADC2_seq2_2_align=Right aligned  ADC2_seq2_2_overSampling=x1 (12 bits)  ADC3_seq2_2_TXT=Not Used  ADC3_seq2_2_align=Right aligned  ADC3_seq2_2_overSampling=x1 (12 bits)  ADC4_seq2_2_TXT=Not Used  ADC4_seq2_2_align=Right aligned  ADC4_seq2_2_overSampling=x1 (12 bits)  ADC5_seq2_2_TXT=Not Used  ADC5_seq2_2_align=Right aligned  ADC5_seq2_2_overSampling=x1 (12 bits)  ADC1_seq2_3_TXT=Not Used  ADC1_seq2_3_align=Right aligned  ADC1_seq2_3_overSampling=x1 (12 bits)  ADC2_seq2_3_TXT=Not Used  ADC2_seq2_3_align=Right aligned  ADC2_seq2_3_overSampling=x1 (12 bits)  ADC3_seq2_3_TXT=Not Used  ADC3_seq2_3_align=Right aligned  ADC3_seq2_3_overSampling=x1 (12 bits)  ADC4_seq2_3_TXT=Not Used  ADC4_seq2_3_align=Right aligned  ADC4_seq2_3_overSampling=x1 (12 bits)  ADC5_seq2_3_TXT=Not Used  ADC5_seq2_3_align=Right aligned  ADC5_seq2_3_overSampling=x1 (12 bits)  ADC1_seq2_4_TXT=Not Used  ADC1_seq2_4_align=Right aligned  ADC1_seq2_4_overSampling=x1 (12 bits)  ADC2_seq2_4_TXT=Not Used  ADC2_seq2_4_align=Right aligned  ADC2_seq2_4_overSampling=x1 (12 bits)  ADC3_seq2_4_TXT=Not Used  ADC3_seq2_4_align=Right aligned  ADC3_seq2_4_overSampling=x1 (12 bits)  ADC4_seq2_4_TXT=Not Used  ADC4_seq2_4_align=Right aligned  ADC4_seq2_4_overSampling=x1 (12 bits)  ADC5_seq2_4_TXT=Not Used  ADC5_seq2_4_align=Right aligned  ADC5_seq2_4_overSampling=x1 (12 bits)  ADC1_seq2_5_TXT=Not Used  ADC1_seq2_5_align=Right aligned  ADC1_seq2_5_overSampling=x1 (12 bits)  ADC2_seq2_5_TXT=Not Used  ADC2_seq2_5_align=Right aligned  ADC2_seq2_5_overSampling=x1 (12 bits)  ADC3_seq2_5_TXT=Not Used  ADC3_seq2_5_align=Right aligned  ADC3_seq2_5_overSampling=x1 (12 bits)  ADC4_seq2_5_TXT=Not Used  ADC4_seq2_5_align=Right aligned  ADC4_seq2_5_overSampling=x1 (12 bits)  ADC5_seq2_5_TXT=Not Used  ADC5_seq2_5_align=Right aligned  ADC5_seq2_5_overSampling=x1 (12 bits)  ADC_TRG2_ACCBRST_seq2=Burst - not interruptible  ADC1_NINSEL_seq2_TXT=Vss - single ended (unsigned)  ADC2_NINSEL_seq2_TXT=Vss - single ended (unsigned)  ADC3_NINSEL_seq2_TXT=Vss - single ended (unsigned)  ADC4_NINSEL_seq2_TXT=Vss - single ended (unsigned)  ADC5_NINSEL_seq2_TXT=Vss - single ended (unsigned)  TrigTimeStep_seq2=off  info_seq2=0  TrigSource_seq3_TXT=after previous sequence  SampleTime_seq3_Tad_TXT="0.5 Tad  = 6.25ns  -  Rin < 0 kOhm"  ADC1_seq3_TXT=Not Used  ADC1_seq3_align=Right aligned  ADC1_seq3_overSampling=x1 (12 bits)  ADC2_seq3_TXT=Not Used  ADC2_seq3_align=Right aligned  ADC2_seq3_overSampling=x1 (12 bits)  ADC3_seq3_TXT=Not Used  ADC3_seq3_align=Right aligned  ADC3_seq3_overSampling=x1 (12 bits)  ADC4_seq3_TXT=Not Used  ADC4_seq3_align=Right aligned  ADC4_seq3_overSampling=x1 (12 bits)  ADC5_seq3_TXT=Not Used  ADC5_seq3_align=Right aligned  ADC5_seq3_overSampling=x1 (12 bits)  ADC1_seq3_1_TXT=Not Used  ADC1_seq3_1_align=Right aligned  ADC1_seq3_1_overSampling=x1 (12 bits)  ADC2_seq3_1_TXT=Not Used  ADC2_seq3_1_align=Right aligned  ADC2_seq3_1_overSampling=x1 (12 bits)  ADC3_seq3_1_TXT=Not Used  ADC3_seq3_1_align=Right aligned  ADC3_seq3_1_overSampling=x1 (12 bits)  ADC4_seq3_1_TXT=Not Used  ADC4_seq3_1_align=Right aligned  ADC4_seq3_1_overSampling=x1 (12 bits)  ADC5_seq3_1_TXT=Not Used  ADC5_seq3_1_align=Right aligned  ADC5_seq3_1_overSampling=x1 (12 bits)  ADC1_seq3_2_TXT=Not Used  ADC1_seq3_2_align=Right aligned  ADC1_seq3_2_overSampling=x1 (12 bits)  ADC2_seq3_2_TXT=Not Used  ADC2_seq3_2_align=Right aligned  ADC2_seq3_2_overSampling=x1 (12 bits)  ADC3_seq3_2_TXT=Not Used  ADC3_seq3_2_align=Right aligned  ADC3_seq3_2_overSampling=x1 (12 bits)  ADC4_seq3_2_TXT=Not Used  ADC4_seq3_2_align=Right aligned  ADC4_seq3_2_overSampling=x1 (12 bits)  ADC5_seq3_2_TXT=Not Used  ADC5_seq3_2_align=Right aligned  ADC5_seq3_2_overSampling=x1 (12 bits)  ADC1_seq3_3_TXT=Not Used  ADC1_seq3_3_align=Right aligned  ADC1_seq3_3_overSampling=x1 (12 bits)  ADC2_seq3_3_TXT=Not Used  ADC2_seq3_3_align=Right aligned  ADC2_seq3_3_overSampling=x1 (12 bits)  ADC3_seq3_3_TXT=Not Used  ADC3_seq3_3_align=Right aligned  ADC3_seq3_3_overSampling=x1 (12 bits)  ADC4_seq3_3_TXT=Not Used  ADC4_seq3_3_align=Right aligned  ADC4_seq3_3_overSampling=x1 (12 bits)  ADC5_seq3_3_TXT=Not Used  ADC5_seq3_3_align=Right aligned  ADC5_seq3_3_overSampling=x1 (12 bits)  ADC1_seq3_4_TXT=Not Used  ADC1_seq3_4_align=Right aligned  ADC1_seq3_4_overSampling=x1 (12 bits)  ADC2_seq3_4_TXT=Not Used  ADC2_seq3_4_align=Right aligned  ADC2_seq3_4_overSampling=x1 (12 bits)  ADC3_seq3_4_TXT=Not Used  ADC3_seq3_4_align=Right aligned  ADC3_seq3_4_overSampling=x1 (12 bits)  ADC4_seq3_4_TXT=Not Used  ADC4_seq3_4_align=Right aligned  ADC4_seq3_4_overSampling=x1 (12 bits)  ADC5_seq3_4_TXT=Not Used  ADC5_seq3_4_align=Right aligned  ADC5_seq3_4_overSampling=x1 (12 bits)  ADC1_seq3_5_TXT=Not Used  ADC1_seq3_5_align=Right aligned  ADC1_seq3_5_overSampling=x1 (12 bits)  ADC2_seq3_5_TXT=Not Used  ADC2_seq3_5_align=Right aligned  ADC2_seq3_5_overSampling=x1 (12 bits)  ADC3_seq3_5_TXT=Not Used  ADC3_seq3_5_align=Right aligned  ADC3_seq3_5_overSampling=x1 (12 bits)  ADC4_seq3_5_TXT=Not Used  ADC4_seq3_5_align=Right aligned  ADC4_seq3_5_overSampling=x1 (12 bits)  ADC5_seq3_5_TXT=Not Used  ADC5_seq3_5_align=Right aligned  ADC5_seq3_5_overSampling=x1 (12 bits)  ADC_TRG2_ACCBRST_seq3=Burst - not interruptible  ADC1_NINSEL_seq3_TXT=Vss - single ended (unsigned)  ADC2_NINSEL_seq3_TXT=Vss - single ended (unsigned)  ADC3_NINSEL_seq3_TXT=Vss - single ended (unsigned)  ADC4_NINSEL_seq3_TXT=Vss - single ended (unsigned)  ADC5_NINSEL_seq3_TXT=Vss - single ended (unsigned)  TrigTimeStep_seq3=off  info_seq3=0  TrigSource_seq4_TXT=after previous sequence  SampleTime_seq4_Tad_TXT="0.5 Tad  = 6.25ns  -  Rin < 0 kOhm"  ADC1_seq4_TXT=Not Used  ADC1_seq4_align=Right aligned  ADC1_seq4_overSampling=x1 (12 bits)  ADC2_seq4_TXT=Not Used  ADC2_seq4_align=Right aligned  ADC2_seq4_overSampling=x1 (12 bits)  ADC3_seq4_TXT=Not Used  ADC3_seq4_align=Right aligned  ADC3_seq4_overSampling=x1 (12 bits)  ADC4_seq4_TXT=Not Used  ADC4_seq4_align=Right aligned  ADC4_seq4_overSampling=x1 (12 bits)  ADC5_seq4_TXT=Not Used  ADC5_seq4_align=Right aligned  ADC5_seq4_overSampling=x1 (12 bits)  ADC1_seq4_1_TXT=Not Used  ADC1_seq4_1_align=Right aligned  ADC1_seq4_1_overSampling=x1 (12 bits)  ADC2_seq4_1_TXT=Not Used  ADC2_seq4_1_align=Right aligned  ADC2_seq4_1_overSampling=x1 (12 bits)  ADC3_seq4_1_TXT=Not Used  ADC3_seq4_1_align=Right aligned  ADC3_seq4_1_overSampling=x1 (12 bits)  ADC4_seq4_1_TXT=Not Used  ADC4_seq4_1_align=Right aligned  ADC4_seq4_1_overSampling=x1 (12 bits)  ADC5_seq4_1_TXT=Not Used  ADC5_seq4_1_align=Right aligned  ADC5_seq4_1_overSampling=x1 (12 bits)  ADC1_seq4_2_TXT=Not Used  ADC1_seq4_2_align=Right aligned  ADC1_seq4_2_overSampling=x1 (12 bits)  ADC2_seq4_2_TXT=Not Used  ADC2_seq4_2_align=Right aligned  ADC2_seq4_2_overSampling=x1 (12 bits)  ADC3_seq4_2_TXT=Not Used  ADC3_seq4_2_align=Right aligned  ADC3_seq4_2_overSampling=x1 (12 bits)  ADC4_seq4_2_TXT=Not Used  ADC4_seq4_2_align=Right aligned  ADC4_seq4_2_overSampling=x1 (12 bits)  ADC5_seq4_2_TXT=Not Used  ADC5_seq4_2_align=Right aligned  ADC5_seq4_2_overSampling=x1 (12 bits)  ADC1_seq4_3_TXT=Not Used  ADC1_seq4_3_align=Right aligned  ADC1_seq4_3_overSampling=x1 (12 bits)  ADC2_seq4_3_TXT=Not Used  ADC2_seq4_3_align=Right aligned  ADC2_seq4_3_overSampling=x1 (12 bits)  ADC3_seq4_3_TXT=Not Used  ADC3_seq4_3_align=Right aligned  ADC3_seq4_3_overSampling=x1 (12 bits)  ADC4_seq4_3_TXT=Not Used  ADC4_seq4_3_align=Right aligned  ADC4_seq4_3_overSampling=x1 (12 bits)  ADC5_seq4_3_TXT=Not Used  ADC5_seq4_3_align=Right aligned  ADC5_seq4_3_overSampling=x1 (12 bits)  ADC1_seq4_4_TXT=Not Used  ADC1_seq4_4_align=Right aligned  ADC1_seq4_4_overSampling=x1 (12 bits)  ADC2_seq4_4_TXT=Not Used  ADC2_seq4_4_align=Right aligned  ADC2_seq4_4_overSampling=x1 (12 bits)  ADC3_seq4_4_TXT=Not Used  ADC3_seq4_4_align=Right aligned  ADC3_seq4_4_overSampling=x1 (12 bits)  ADC4_seq4_4_TXT=Not Used  ADC4_seq4_4_align=Right aligned  ADC4_seq4_4_overSampling=x1 (12 bits)  ADC5_seq4_4_TXT=Not Used  ADC5_seq4_4_align=Right aligned  ADC5_seq4_4_overSampling=x1 (12 bits)  ADC1_seq4_5_TXT=Not Used  ADC1_seq4_5_align=Right aligned  ADC1_seq4_5_overSampling=x1 (12 bits)  ADC2_seq4_5_TXT=Not Used  ADC2_seq4_5_align=Right aligned  ADC2_seq4_5_overSampling=x1 (12 bits)  ADC3_seq4_5_TXT=Not Used  ADC3_seq4_5_align=Right aligned  ADC3_seq4_5_overSampling=x1 (12 bits)  ADC4_seq4_5_TXT=Not Used  ADC4_seq4_5_align=Right aligned  ADC4_seq4_5_overSampling=x1 (12 bits)  ADC5_seq4_5_TXT=Not Used  ADC5_seq4_5_align=Right aligned  ADC5_seq4_5_overSampling=x1 (12 bits)  ADC_TRG2_ACCBRST_seq4=Burst - not interruptible  ADC1_NINSEL_seq4_TXT=Vss - single ended (unsigned)  ADC2_NINSEL_seq4_TXT=Vss - single ended (unsigned)  ADC3_NINSEL_seq4_TXT=Vss - single ended (unsigned)  ADC4_NINSEL_seq4_TXT=Vss - single ended (unsigned)  ADC5_NINSEL_seq4_TXT=Vss - single ended (unsigned)  TrigTimeStep_seq4=off  info_seq4=0  TrigSource_seq5_TXT=after previous sequence  SampleTime_seq5_Tad_TXT="0.5 Tad  = 6.25ns  -  Rin < 0 kOhm"  ADC1_seq5_TXT=Not Used  ADC1_seq5_align=Right aligned  ADC1_seq5_overSampling=x1 (12 bits)  ADC2_seq5_TXT=Not Used  ADC2_seq5_align=Right aligned  ADC2_seq5_overSampling=x1 (12 bits)  ADC3_seq5_TXT=Not Used  ADC3_seq5_align=Right aligned  ADC3_seq5_overSampling=x1 (12 bits)  ADC4_seq5_TXT=Not Used  ADC4_seq5_align=Right aligned  ADC4_seq5_overSampling=x1 (12 bits)  ADC5_seq5_TXT=Not Used  ADC5_seq5_align=Right aligned  ADC5_seq5_overSampling=x1 (12 bits)  ADC1_seq5_1_TXT=Not Used  ADC1_seq5_1_align=Right aligned  ADC1_seq5_1_overSampling=x1 (12 bits)  ADC2_seq5_1_TXT=Not Used  ADC2_seq5_1_align=Right aligned  ADC2_seq5_1_overSampling=x1 (12 bits)  ADC3_seq5_1_TXT=Not Used  ADC3_seq5_1_align=Right aligned  ADC3_seq5_1_overSampling=x1 (12 bits)  ADC4_seq5_1_TXT=Not Used  ADC4_seq5_1_align=Right aligned  ADC4_seq5_1_overSampling=x1 (12 bits)  ADC5_seq5_1_TXT=Not Used  ADC5_seq5_1_align=Right aligned  ADC5_seq5_1_overSampling=x1 (12 bits)  ADC1_seq5_2_TXT=Not Used  ADC1_seq5_2_align=Right aligned  ADC1_seq5_2_overSampling=x1 (12 bits)  ADC2_seq5_2_TXT=Not Used  ADC2_seq5_2_align=Right aligned  ADC2_seq5_2_overSampling=x1 (12 bits)  ADC3_seq5_2_TXT=Not Used  ADC3_seq5_2_align=Right aligned  ADC3_seq5_2_overSampling=x1 (12 bits)  ADC4_seq5_2_TXT=Not Used  ADC4_seq5_2_align=Right aligned  ADC4_seq5_2_overSampling=x1 (12 bits)  ADC5_seq5_2_TXT=Not Used  ADC5_seq5_2_align=Right aligned  ADC5_seq5_2_overSampling=x1 (12 bits)  ADC1_seq5_3_TXT=Not Used  ADC1_seq5_3_align=Right aligned  ADC1_seq5_3_overSampling=x1 (12 bits)  ADC2_seq5_3_TXT=Not Used  ADC2_seq5_3_align=Right aligned  ADC2_seq5_3_overSampling=x1 (12 bits)  ADC3_seq5_3_TXT=Not Used  ADC3_seq5_3_align=Right aligned  ADC3_seq5_3_overSampling=x1 (12 bits)  ADC4_seq5_3_TXT=Not Used  ADC4_seq5_3_align=Right aligned  ADC4_seq5_3_overSampling=x1 (12 bits)  ADC5_seq5_3_TXT=Not Used  ADC5_seq5_3_align=Right aligned  ADC5_seq5_3_overSampling=x1 (12 bits)  ADC1_seq5_4_TXT=Not Used  ADC1_seq5_4_align=Right aligned  ADC1_seq5_4_overSampling=x1 (12 bits)  ADC2_seq5_4_TXT=Not Used  ADC2_seq5_4_align=Right aligned  ADC2_seq5_4_overSampling=x1 (12 bits)  ADC3_seq5_4_TXT=Not Used  ADC3_seq5_4_align=Right aligned  ADC3_seq5_4_overSampling=x1 (12 bits)  ADC4_seq5_4_TXT=Not Used  ADC4_seq5_4_align=Right aligned  ADC4_seq5_4_overSampling=x1 (12 bits)  ADC5_seq5_4_TXT=Not Used  ADC5_seq5_4_align=Right aligned  ADC5_seq5_4_overSampling=x1 (12 bits)  ADC1_seq5_5_TXT=Not Used  ADC1_seq5_5_align=Right aligned  ADC1_seq5_5_overSampling=x1 (12 bits)  ADC2_seq5_5_TXT=Not Used  ADC2_seq5_5_align=Right aligned  ADC2_seq5_5_overSampling=x1 (12 bits)  ADC3_seq5_5_TXT=Not Used  ADC3_seq5_5_align=Right aligned  ADC3_seq5_5_overSampling=x1 (12 bits)  ADC4_seq5_5_TXT=Not Used  ADC4_seq5_5_align=Right aligned  ADC4_seq5_5_overSampling=x1 (12 bits)  ADC5_seq5_5_TXT=Not Used  ADC5_seq5_5_align=Right aligned  ADC5_seq5_5_overSampling=x1 (12 bits)  ADC_TRG2_ACCBRST_seq5=Burst - not interruptible  ADC1_NINSEL_seq5_TXT=Vss - single ended (unsigned)  ADC2_NINSEL_seq5_TXT=Vss - single ended (unsigned)  ADC3_NINSEL_seq5_TXT=Vss - single ended (unsigned)  ADC4_NINSEL_seq5_TXT=Vss - single ended (unsigned)  ADC5_NINSEL_seq5_TXT=Vss - single ended (unsigned)  TrigTimeStep_seq5=off  info_seq5=0
      settings: SourceProductName=MPLAB Device Blocks for Simulink
  Ia : Outport  VectorParamsAs1DForOutWhenUnconnected=off
  Ib : Outport  Port=2  VectorParamsAs1DForOutWhenUnconnected=off
  IBus : Outport  Port=3  VectorParamsAs1DForOutWhenUnconnected=off
  Pot : Outport  Port=4  VectorParamsAs1DForOutWhenUnconnected=off
  V_BUS : Outport  Port=5  VectorParamsAs1DForOutWhenUnconnected=off
  Va : Outport  Port=6  VectorParamsAs1DForOutWhenUnconnected=off
  Vb : Outport  Port=7  VectorParamsAs1DForOutWhenUnconnected=off
  Vc : Outport  Port=8  VectorParamsAs1DForOutWhenUnconnected=off
  wires:
  ADC HS 12b dsPICA1/5 -> Vc/1
  ADC HS 12b dsPICA1/3 -> Vb/1
  ADC HS 12b dsPICA1/4 -> Va/1
  ADC HS 12b dsPICA1/1 -> Ia/1
  ADC HS 12b dsPICA1/2 -> Ib/1
  ADC HS 12b dsPICA2/2 -> V_BUS/1
  ADC HS 12b dsPICA2/1 -> IBus/1
  ADC HS 12b dsPICA2/3 -> Pot/1

== system MCU_vectorControl_dsPIC33AK128MC106_MCLV_48V_300W_Float/BOARD MCLV-48V-300W dsPIC33AK128MC106 MC DIM/Center & sign reversal ==
  Iab : Inport
  Bias Update : Inport  Port=2
  Cast : DataTypeConversion  OutDataTypeStr=single  SaturateOnIntegerOverflow=off  RndMeth=Floor
  LPF : Subsystem
  Sum : Sum  Inputs=+-
  Out1 : Outport
  wires:
  Sum/1 -> Out1/1
  Iab/1 -> Cast/1
  Bias Update/1 -> LPF/Enable
  Cast/1 -> Sum/2, LPF/1(U)
  LPF/1(Y) -> Sum/1

== system MCU_vectorControl_dsPIC33AK128MC106_MCLV_48V_300W_Float/BOARD MCLV-48V-300W dsPIC33AK128MC106 MC DIM/Downsample Averaged x20 ==
  note: DownSample & Average by changing data scaling
  In1 : Inport
  Compare To Constant : simulink/Logic and Bit Operations/Compare To Constant  relop===  const=1  OutDataTypeStr=boolean
  Counter Limited : simulink/Sources/Counter Limited  uplimit=DownSample-1  tsamp=-1
  Data Type Duplicate : DataTypeDuplicate
  Data Type Propagation : simulink/Signal Attributes/Data Type Propagation  PropDataType=fixdt(1, 16)  IfRefDouble=double  IfRefSingle=single  IsSigned=IsSigned1 or IsSigned2  NumBitsBase=NumBits1+NumBits2  NumBitsMult=1  NumBitsAdd=0  NumBitsAllowFinal=-1  PropScaling=2^-10  ValuesUsedBestPrec=[5 -7]  SlopeBase=Slope1  SlopeMult=1  SlopeAdd=0  BiasBase=Bias1  BiasMult=1  BiasAdd=0
  Discrete-Time Integrator : DiscreteIntegrator  IntegratorMethod=Accumulation: Backward Euler  gainval=1  ExternalReset=sampled level  SampleTime=-1  OutDataTypeStr=Inherit: Inherit via back propagation  ICPrevOutput=DiscIntNeverNeededParam  ICPrevScaledInput=DiscIntNeverNeededParam
  Gain : Gain  Gain=1/DownSample  OutDataTypeStr=Inherit: Inherit via back propagation  RndMeth=Round
  Rate Transition1 : RateTransition  OutPortSampleTimeOpt=Multiple of input port sample time  OutPortSampleTimeMultiple=DownSample  OutPortSampleTime=DownSample
  Rate Transition3 : RateTransition  OutPortSampleTimeOpt=Multiple of input port sample time  OutPortSampleTimeMultiple=DownSample  OutPortSampleTime=DownSample
  Out1 : Outport  VectorParamsAs1DForOutWhenUnconnected=off
  wires:
  Rate Transition3/1 -> Gain/1
  In1/1 -> Rate Transition1/1, Discrete-Time Integrator/1, Data Type Propagation/2, Data Type Propagation/1
  Compare To Constant/1 -> Discrete-Time Integrator/2
  Discrete-Time Integrator/1 -> Data Type Propagation/3, Rate Transition3/1
  Counter Limited/1 -> Compare To Constant/1
  Gain/1 -> Data Type Duplicate/2, Out1/1
  Rate Transition1/1 -> Data Type Duplicate/1

== system MCU_vectorControl_dsPIC33AK128MC106_MCLV_48V_300W_Float/BOARD MCLV-48V-300W dsPIC33AK128MC106 MC DIM/Downsample x20 ==
  note: DownSample & Average by changing data scaling
  In1 : Inport
  Compare To Constant : simulink/Logic and Bit Operations/Compare To Constant  relop===  const=1  OutDataTypeStr=boolean
  Counter Limited : simulink/Sources/Counter Limited  uplimit=DownSample-1  tsamp=-1
  Data Type Duplicate : DataTypeDuplicate
  Data Type Propagation : simulink/Signal Attributes/Data Type Propagation  PropDataType=fixdt(1, 16)  IfRefDouble=double  IfRefSingle=single  IsSigned=IsSigned1 or IsSigned2  NumBitsBase=NumBits1+NumBits2  NumBitsMult=1  NumBitsAdd=0  NumBitsAllowFinal=-1  PropScaling=2^-10  ValuesUsedBestPrec=[5 -7]  SlopeBase=Slope1  SlopeMult=1  SlopeAdd=0  BiasBase=Bias1  BiasMult=1  BiasAdd=0
  Discrete-Time Integrator : DiscreteIntegrator  IntegratorMethod=Accumulation: Backward Euler  gainval=1  ExternalReset=sampled level  SampleTime=-1  OutDataTypeStr=Inherit: Inherit via back propagation  ICPrevOutput=DiscIntNeverNeededParam  ICPrevScaledInput=DiscIntNeverNeededParam
  Gain : Gain  Gain=1/DownSample  OutDataTypeStr=Inherit: Inherit via back propagation  RndMeth=Round
  Rate Transition1 : RateTransition  OutPortSampleTimeOpt=Multiple of input port sample time  OutPortSampleTimeMultiple=DownSample  OutPortSampleTime=DownSample
  Rate Transition3 : RateTransition  OutPortSampleTimeOpt=Multiple of input port sample time  OutPortSampleTimeMultiple=DownSample  OutPortSampleTime=DownSample
  Out1 : Outport  VectorParamsAs1DForOutWhenUnconnected=off
  wires:
  Rate Transition1/1 -> Data Type Duplicate/1
  Gain/1 -> Out1/1, Data Type Duplicate/2
  Counter Limited/1 -> Compare To Constant/1
  Discrete-Time Integrator/1 -> Rate Transition3/1, Data Type Propagation/3
  Compare To Constant/1 -> Discrete-Time Integrator/2
  In1/1 -> Data Type Propagation/1, Data Type Propagation/2, Discrete-Time Integrator/1, Rate Transition1/1
  Rate Transition3/1 -> Gain/1
